simulink model "LCK_0112"  (R2018b)
settings: Solver=FixedStepDiscrete  StartTime=0.0  StopTime=inf  FixedStep=0.01  RelTol=1e-3
PostLoadFcn:
  | if any(exist('dsrtsu_mdlpostloadfcn', 'file') ~= 0), dsrtsu_mdlpostloadfcn('Execute', bdroot); end
values from neighbouring files (symbols this model uses):
  C_DEG2RAD = 0.0175    [LCK_Macro.sldd]
  C_KPH2MPS = 0.2778    [LCK_Macro.sldd]
  C_NEARZERO = 0.0001    [LCK_Macro.sldd]
  C_ONE = 1.0    [LCK_Macro.sldd]
  C_RAD2DEG = 57.2958    [LCK_Macro.sldd]
  C_ZERO = 0.0    [LCK_Macro.sldd]
  k_accel_pedal_pos_per_speed_x : value not decoded    [LCK_LogicPara.sldd]
  k_accel_pedal_pos_per_speed_z : value not decoded    [LCK_LogicPara.sldd]
  k_brake_suprress_hold = 1000.0    [LCK_LogicPara.sldd]
  k_driver_appl_torque_filt = 50.0    [LCK_LogicPara.sldd]
  k_driver_suppression_hold_time = 3000.0    [LCK_LogicPara.sldd]
  k_hands_on_wheel_hold_msec = 500.0    [LCK_LogicPara.sldd]
  k_hands_on_wheel_torque_hi = 0.2    [LCK_LogicPara.sldd]
  k_hands_on_wheel_torque_lo = 0.15    [LCK_LogicPara.sldd]
  k_handsoff_delay_cycles = 50.0    [LCK_LogicPara.sldd]
  k_handsoff_torq_Lo_CR = 0.3    [LCK_LogicPara.sldd]
  k_handson_delay_cycles = 5.0    [LCK_LogicPara.sldd]
  k_HighAccel_suppress_hold = 3000.0    [LCK_LogicPara.sldd]
  k_HLR_suprress_hold = 3000.0    [LCK_LogicPara.sldd]
  k_hs_StrAng_CR_threshold_z : value not decoded    [LCK_LogicPara.sldd]
  k_LC_Exit_Switch = 0.0    [LCK_LogicPara.sldd]
  k_LCG_Configured = 1.0    [LCK_LogicPara.sldd]
  k_LCK_A0_Rdy2Act_UseConst = 0.0    [LCK_LogicPara.sldd]
  k_LCK_A0Fac_ActSta : value not decoded    [LCK_CtrlPara.sldd]
  k_LCK_A0Fac_DrvStm : value not decoded    [LCK_CtrlPara.sldd]
  k_LCK_A0Shift_LftCurv : value not decoded    [LCK_CtrlPara.sldd]
  k_LCK_A0Shift_RgtCurv : value not decoded    [LCK_CtrlPara.sldd]
  k_LCK_A0Shift_StraLan = 0.0    [LCK_CtrlPara.sldd]
  k_LCK_A0ShiftFac_Dy_LftCurv : value not decoded    [LCK_CtrlPara.sldd]
  k_LCK_A0ShiftFac_Dy_RgtCurv : value not decoded    [LCK_CtrlPara.sldd]
  k_LCK_A0ShiftFac_Vspd : value not decoded    [LCK_CtrlPara.sldd]
  k_LCK_accel_inhibit_thold = 35.0    [LCK_LogicPara.sldd]
  k_LCK_Active2Ready_Mask = 255.0    [LCK_LogicPara.sldd]
  k_LCK_CvatRateBks : value not decoded    [LCK_CtrlPara.sldd]
  k_LCK_CvatrBks : value not decoded    [LCK_CtrlPara.sldd]
  k_LCK_DFac_Dy : value not decoded    [LCK_CtrlPara.sldd]
  k_LCK_DFac_Dy_Curv : value not decoded    [LCK_CtrlPara.sldd]
  k_LCK_DFac_HaCurCen : value not decoded    [LCK_CtrlPara.sldd]
  k_LCK_DFac_HaCurSid : value not decoded    [LCK_CtrlPara.sldd]
  k_LCK_DFac_HadCurCen : value not decoded    [LCK_CtrlPara.sldd]
  k_LCK_DFac_HadCurSid : value not decoded    [LCK_CtrlPara.sldd]
  k_LCK_DFac_HadStrCen : value not decoded    [LCK_CtrlPara.sldd]
  k_LCK_DFac_HadStrSid : value not decoded    [LCK_CtrlPara.sldd]
  k_LCK_DFac_HaStrCen : value not decoded    [LCK_CtrlPara.sldd]
  k_LCK_DFac_HaStrSid : value not decoded    [LCK_CtrlPara.sldd]
  k_LCK_DFac_Rad : value not decoded    [LCK_CtrlPara.sldd]
  k_LCK_DFac_SA_CurCen : value not decoded    [LCK_CtrlPara.sldd]
  k_LCK_DFac_SA_CurSid : value not decoded    [LCK_CtrlPara.sldd]
  k_LCK_DFac_SA_StrCen : value not decoded    [LCK_CtrlPara.sldd]
  k_LCK_DFac_SA_StrSid : value not decoded    [LCK_CtrlPara.sldd]
  k_LCK_DFac_SS_CurCen : value not decoded    [LCK_CtrlPara.sldd]
  k_LCK_DFac_SS_CurSid : value not decoded    [LCK_CtrlPara.sldd]
  k_LCK_DFac_SS_StrCen : value not decoded    [LCK_CtrlPara.sldd]
  k_LCK_DFac_SS_StrSid : value not decoded    [LCK_CtrlPara.sldd]
  k_LCK_DFac_Vspd : value not decoded    [LCK_CtrlPara.sldd]
  k_LCK_DlyTm_DrvStim = 0.2    [LCK_CtrlPara.sldd]
  k_LCK_DTermMax = 2.0    [LCK_CtrlPara.sldd]
  k_LCK_DyBks_Curv : value not decoded    [LCK_CtrlPara.sldd]
  k_LCK_Enable_POOnly = 1.0    [LCK_LogicPara.sldd]
  k_LCK_Entry_DistBuffer = 0.1    [LCK_LogicPara.sldd]
  k_LCK_Fac_Vspd2RngThr_FalRec = 0.23    [LCK_CtrlPara.sldd]
  k_LCK_Ffw_CvatSwh = 0.0    [LCK_CtrlPara.sldd]
  k_LCK_Ffw_DyBks : value not decoded    [LCK_CtrlPara.sldd]
  k_LCK_Ffw_TimCon_CmdFlt = 0.0    [LCK_CtrlPara.sldd]
  k_LCK_FfwDeltaFac_Rad_Lft : value not decoded    [LCK_CtrlPara.sldd]
  k_LCK_FfwDeltaFac_Rad_Rgt : value not decoded    [LCK_CtrlPara.sldd]
  k_LCK_FfwDeltaFac_Vspd : value not decoded    [LCK_CtrlPara.sldd]
  k_LCK_FfwFac_CvatRate_Lft : value not decoded    [LCK_CtrlPara.sldd]
  k_LCK_FfwFac_CvatRate_Rgt : value not decoded    [LCK_CtrlPara.sldd]
  k_LCK_FfwFac_Dy : value not decoded    [LCK_CtrlPara.sldd]
  k_LCK_FfwFac_Rad_Lft : value not decoded    [LCK_CtrlPara.sldd]
  k_LCK_FfwFac_Rad_Rgt : value not decoded    [LCK_CtrlPara.sldd]
  k_LCK_FfwFac_Vspd : value not decoded    [LCK_CtrlPara.sldd]
  k_LCK_FfwTorq_Cvat : value not decoded    [LCK_CtrlPara.sldd]
  k_LCK_HAFac_ActSta : value not decoded    [LCK_CtrlPara.sldd]
  k_LCK_HAFac_DrvStm : value not decoded    [LCK_CtrlPara.sldd]
  k_LCK_HaloTime = 2000.0    [LCK_LogicPara.sldd]
  k_LCK_HaloTime_Switch = 0.0    [LCK_LogicPara.sldd]
  k_LCK_HARFac_ActSta : value not decoded    [LCK_CtrlPara.sldd]
  k_LCK_HARFac_DrvStm : value not decoded    [LCK_CtrlPara.sldd]
  k_LCK_Hed_DyBks : value not decoded    [LCK_CtrlPara.sldd]
  k_LCK_HedAngDiffX : value not decoded    [LCK_CtrlPara.sldd]
  k_LCK_HedAngRateDiffX : value not decoded    [LCK_CtrlPara.sldd]
  k_LCK_HndsOnWhel_DlyTm_Idl2Rdy = 0.0    [LCK_LogicPara.sldd]
  k_LCK_host_veh_width = 1.86    [LCK_LogicPara.sldd]
  k_LCK_Idle2Ready_Mask = 239.0    [LCK_LogicPara.sldd]
  k_LCK_Junc_SusTime = 1.0    [LCK_LogicPara.sldd]
  k_LCK_KpKdDecSlopeLmt = 10.0    [LCK_CtrlPara.sldd]
  k_LCK_KpKdIncSlopeLmt = 5.0    [LCK_CtrlPara.sldd]
  k_LCK_Lat_Ctrl_DFac_Lft = 1.0    [LCK_CtrlPara.sldd]
  k_LCK_Lat_Ctrl_DFac_Rgt = 1.05    [LCK_CtrlPara.sldd]
  k_LCK_Lat_Ctrl_Kd = 0.8    [LCK_CtrlPara.sldd]
  k_LCK_Lat_Ctrl_Ki = 0.5    [LCK_CtrlPara.sldd]
  k_LCK_Lat_Ctrl_Kp = 0.7    [LCK_CtrlPara.sldd]
  k_LCK_Lat_Ctrl_Kp_NearGain = 0.7    [LCK_CtrlPara.sldd]
  k_LCK_Lat_Ctrl_PFac_Lft = 1.0    [LCK_CtrlPara.sldd]
  k_LCK_Lat_Ctrl_PFac_Rgt = 1.05    [LCK_CtrlPara.sldd]
  k_LCK_Lat_Ctrl_TimCon_CmdFlt = 5.0    [LCK_CtrlPara.sldd]
  k_LCK_Lat_DFac_Rad : value not decoded    [LCK_CtrlPara.sldd]
  k_LCK_Lat_DFac_SS_Cur : value not decoded    [LCK_CtrlPara.sldd]
  k_LCK_Lat_DFac_SS_Str : value not decoded    [LCK_CtrlPara.sldd]
  k_LCK_Lat_DFac_Vspd : value not decoded    [LCK_CtrlPara.sldd]
  k_LCK_Lat_DyBks : value not decoded    [LCK_CtrlPara.sldd]
  k_LCK_Lat_IFac_Rad : value not decoded    [LCK_CtrlPara.sldd]
  k_LCK_Lat_IFac_Vspd : value not decoded    [LCK_CtrlPara.sldd]
  k_LCK_Lat_ILmtFac_Dy_CurvLan : value not decoded    [LCK_CtrlPara.sldd]
  k_LCK_Lat_ILmtFac_Dy_StraLan : value not decoded    [LCK_CtrlPara.sldd]
  k_LCK_Lat_ILmtFac_Rad : value not decoded    [LCK_CtrlPara.sldd]
  k_LCK_Lat_ILmtFac_Rad_NearGain = 1.0    [LCK_CtrlPara.sldd]
  k_LCK_Lat_ILmtFac_Vspd_CurvLan : value not decoded    [LCK_CtrlPara.sldd]
  k_LCK_Lat_ILmtFac_Vspd_StraLan : value not decoded    [LCK_CtrlPara.sldd]
  k_LCK_Lat_ITermLmt_Dy = 1.0    [LCK_CtrlPara.sldd]
  k_LCK_Lat_KpKdDecSlopeLmt = 10.0    [LCK_CtrlPara.sldd]
  k_LCK_Lat_KpKdIncSlopeLmt = 10.0    [LCK_CtrlPara.sldd]
  k_LCK_Lat_PFac_Dy_InnLftCur : value not decoded    [LCK_CtrlPara.sldd]
  k_LCK_Lat_PFac_Dy_InnRgtCur : value not decoded    [LCK_CtrlPara.sldd]
  k_LCK_Lat_PFac_Dy_OutLftCur : value not decoded    [LCK_CtrlPara.sldd]
  k_LCK_Lat_PFac_Dy_OutRgtCur : value not decoded    [LCK_CtrlPara.sldd]
  k_LCK_Lat_PFac_Dy_Str : value not decoded    [LCK_CtrlPara.sldd]
  k_LCK_Lat_PFac_Rad : value not decoded    [LCK_CtrlPara.sldd]
  ... (+153 more)
undefined symbols (not defined in the file or in its folder): k_LCK_CurvBks, K_LCK_SPA0A1A2_LMRngCmp_y
libraries: LateralControl_fcns_lib x58, simulink x24
(part 27 of 45)

== system LCK_0112/Lateral_Control_Module/LCK_State_Ctrl/LCK_Mode_Transition/Det_LCK_Switch ==
  LDWLKASwReq : Inport
  Constant6 : Constant  Tag={'output',{'type','Int32'},'date',737184.60397266201}  Description=_GWMAB30P2.LCK.000_1069_  Value=4
  Relational Operator : RelationalOperator  Operator=<=  OutDataTypeStr=boolean  RndMeth=Simplest
  LCK_Switch : Outport
  wires:
  Constant6/1 -> Relational Operator/2
  Relational Operator/1 -> LCK_Switch/1
  LDWLKASwReq/1 -> Relational Operator/1

== system LCK_0112/Lateral_Control_Module/LCK_State_Ctrl/LCK_Mode_Transition/Det_TJA_Lat_Req ==
  TJA_State : Inport
  ZOP_LCK_Activate : Inport  Port=2
  Chart : Stateflow chart  TreatAsAtomicUnit=on
  Constant1 : Constant  Tag={'output',{'type','Int32'},'date',737184.60397266201}  Description=_GWMAB30P2.LCK.000_1069_
  Data Type Conversion89 : DataTypeConversion  Description=_GACA26P4.LCK.000_14_  OutDataTypeStr=boolean
  Logical Operator : Logic  Operator=OR  AllPortsSameDT=off  OutDataTypeStr=boolean
  Relational Operator1 : RelationalOperator  Operator===  OutDataTypeStr=boolean  RndMeth=Simplest
  TJA_Lat_Req : Outport
  wires:
  TJA_State/1 -> Chart/1(TJA_State)
  Constant1/1 -> Relational Operator1/2
  ZOP_LCK_Activate/1 -> Relational Operator1/1
  Logical Operator/1 -> TJA_Lat_Req/1
  Chart/1(TJA_Lat_Req) -> Data Type Conversion89/1
  Relational Operator1/1 -> Logical Operator/2
  Data Type Conversion89/1 -> Logical Operator/1

== system LCK_0112/Lateral_Control_Module/LCK_State_Ctrl/LCK_Mode_Transition/Determination_of_ACTIVE2OFF ==
  TJA_Switch : Inport
  LCK_Switch : Inport  Port=2
  Logical Operator3 : Logic  Tag={'date',737184.60397805553}  Description=_GWMAB30P2.LCK.000_1110_  Operator=NOR  AllPortsSameDT=off  OutDataTypeStr=boolean
  ACTIVE2OFF : Outport
  wires:
  Logical Operator3/1 -> ACTIVE2OFF/1
  LCK_Switch/1 -> Logical Operator3/2
  TJA_Switch/1 -> Logical Operator3/1

== system LCK_0112/Lateral_Control_Module/LCK_State_Ctrl/LCK_Mode_Transition/Determination_of_ERROR2IDLE ==
  ERROR_CONDITION : Inport
  TJA_Switch : Inport  Port=2
  LCK_Switch : Inport  Port=3
  Logical Operator35 : Logic  Tag={'date',737184.60397880792}  Description=_GWMAB30P2.LCK.000_1116_  AllPortsSameDT=off  OutDataTypeStr=boolean
  Logical Operator36 : Logic  Tag={'date',737184.603978912}  Description=_GWMAB30P2.LCK.000_1117_  Operator=OR  AllPortsSameDT=off  OutDataTypeStr=boolean
  Relational Operator40 : RelationalOperator  Tag={'date',737184.6039850926}  Description=_GWMAB30P2.LCK.000_1167_  Operator=~=  OutDataTypeStr=boolean  RndMeth=Nearest
  Relational Operator41 : RelationalOperator  Tag={'date',737184.60398521996}  Description=_GWMAB30P2.LCK.000_1168_  Operator===  OutDataTypeStr=boolean  RndMeth=Nearest
  Relational Operator42 : RelationalOperator  Tag={'date',737184.6039853472}  Description=_GWMAB30P2.LCK.000_1169_  Operator===  OutDataTypeStr=boolean  RndMeth=Nearest
  const26 : Constant  Tag={'output',{'type','Int32'},'date',737184.60399236111}  Description=_GWMAB30P2.LCK.000_1218_
  const27 : Constant  Tag={'output',{'type','Int32'},'date',737184.60399249999}  Description=_GWMAB30P2.LCK.000_1219_
  const28 : Constant  Tag={'output',{'type','Int32'},'date',737184.60399262735}  Description=_GWMAB30P2.LCK.000_1220_
  ERROR2IDLE : Outport
  wires:
  Logical Operator36/1 -> Logical Operator35/2
  ERROR_CONDITION/1 -> Relational Operator40/1
  Relational Operator42/1 -> Logical Operator36/2
  const27/1 -> Relational Operator41/2
  Relational Operator40/1 -> Logical Operator35/1
  const28/1 -> Relational Operator42/2
  Logical Operator35/1 -> ERROR2IDLE/1
  const26/1 -> Relational Operator40/2
  Relational Operator41/1 -> Logical Operator36/1
  LCK_Switch/1 -> Relational Operator42/1
  TJA_Switch/1 -> Relational Operator41/1

== system LCK_0112/Lateral_Control_Module/LCK_State_Ctrl/LCK_Mode_Transition/Determination_of_ERROR2OFF ==
  TJA_Switch : Inport
  LCK_Switch : Inport  Port=2
  Logical Operator3 : Logic  Tag={'date',737184.60397805553}  Description=_GWMAB30P2.LCK.000_1110_  Operator=NOR  AllPortsSameDT=off  OutDataTypeStr=boolean
  ERROR2OFF : Outport
  wires:
  TJA_Switch/1 -> Logical Operator3/1
  LCK_Switch/1 -> Logical Operator3/2
  Logical Operator3/1 -> ERROR2OFF/1

== system LCK_0112/Lateral_Control_Module/LCK_State_Ctrl/LCK_Mode_Transition/Determination_of_ERROR2READY ==
  ERROR2IDLE : Inport
  IDLE2READY : Inport  Port=2
  Logical Operator16 : Logic  Tag={'date',737292.69766146992}  Description=_GWMAB30P4.LCK.000_177_  AllPortsSameDT=off  OutDataTypeStr=boolean
  ERROR2READY : Outport
  wires:
  ERROR2IDLE/1 -> Logical Operator16/1
  IDLE2READY/1 -> Logical Operator16/2
  Logical Operator16/1 -> ERROR2READY/1

== system LCK_0112/Lateral_Control_Module/LCK_State_Ctrl/LCK_Mode_Transition/Determination_of_IDLE2OFF ==
  TJA_Switch : Inport
  LCK_Switch : Inport  Port=2
  Logical Operator3 : Logic  Tag={'date',737184.60397805553}  Description=_GWMAB30P2.LCK.000_1110_  Operator=NOR  AllPortsSameDT=off  OutDataTypeStr=boolean
  IDLE2OFF : Outport
  wires:
  Logical Operator3/1 -> IDLE2OFF/1
  LCK_Switch/1 -> Logical Operator3/2
  TJA_Switch/1 -> Logical Operator3/1
